simulink model "Projet_RST_sim_LIMA_MILITAO_PINHEIRO"  (R2019a)
settings: Solver=VariableStepAuto  StartTime=0.0  StopTime=10.0  FixedStep=1e-6  RelTol=1e-3
undefined symbols (not defined in the file): Am_omega, Bm_omega, den, G_den_RST, G_num_RST, numG2, R, S, T, Te, tsim
settings Model: Creator=dougl  LastModifiedBy=dougl
settings DebuggingCC: UnconnectedInputMsg=none  UnconnectedOutputMsg=none  UnconnectedLineMsg=none  SFMachineParentedDataDiag=error

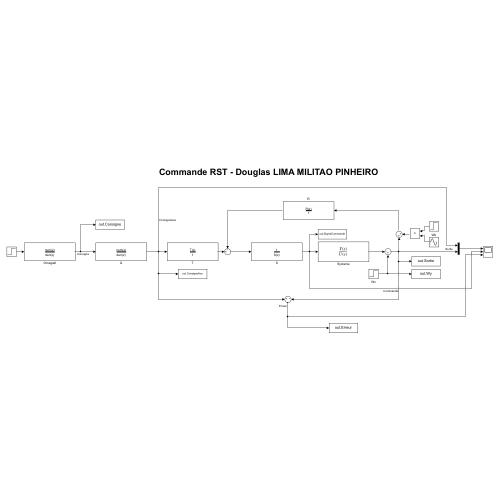
[thumbnail: Simulink's stored preview of the top-level diagram]
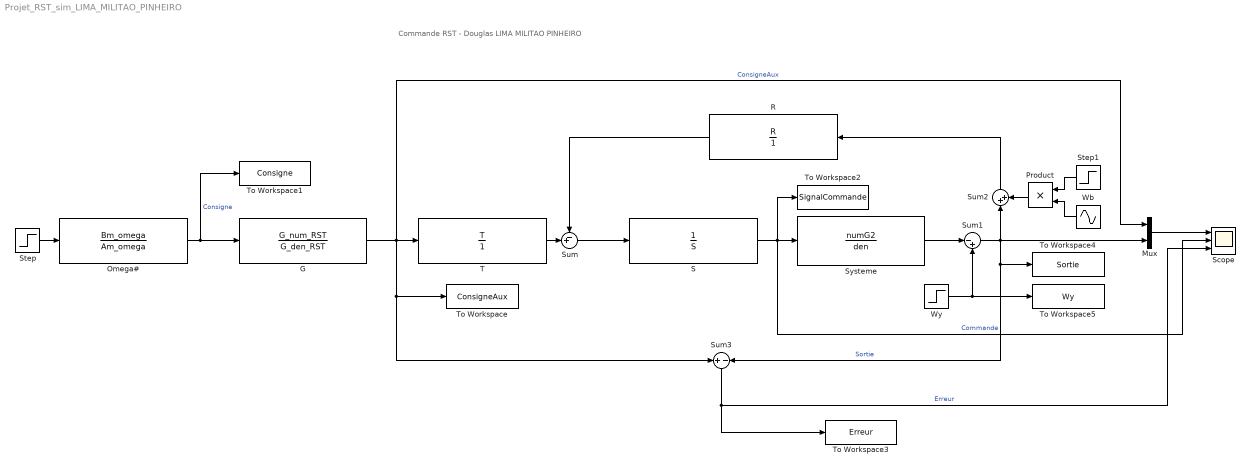
== system Projet_RST_sim_LIMA_MILITAO_PINHEIRO ==
  note: Commande RST - Douglas LIMA MILITAO PINHEIRO
  G : DiscreteFilter  Numerator=G_num_RST  Denominator=G_den_RST  SampleTime=Te
  Mux : Mux  Inputs=2
  Omega# : DiscreteFilter  Numerator=Bm_omega  Denominator=Am_omega  SampleTime=Te
  Product : Product
  R : DiscreteFilter  Numerator=R  Denominator=1  SampleTime=Te
  S : DiscreteFilter  Numerator=1  Denominator=S  SampleTime=Te
  Scope : Scope  NumInputPorts=3
  Step : Step  After=5  SampleTime=0
  Step1 : Step  Time=7  SampleTime=0
  Sum : Sum  Inputs=-+|
  Sum1 : Sum  Inputs=|-+
  Sum2 : Sum  Inputs=|++
  Sum3 : Sum  Inputs=+|-
  Systeme : TransferFcn  Numerator=numG2  Denominator=den
  T : DiscreteFilter  Numerator=T  Denominator=1  SampleTime=Te
  To Workspace : ToWorkspace  VariableName=ConsigneAux  SampleTime=tsim
  To Workspace1 : ToWorkspace  VariableName=Consigne  SampleTime=tsim
  To Workspace2 : ToWorkspace  VariableName=SignalCommande  SampleTime=tsim
  To Workspace3 : ToWorkspace  VariableName=Erreur  SampleTime=tsim
  To Workspace4 : ToWorkspace  VariableName=Sortie  SampleTime=tsim
  To Workspace5 : ToWorkspace  VariableName=Wy  SampleTime=tsim
  Wb : Sin  Amplitude=3  Frequency=2*pi*10  SampleTime=0
  Wy : Step  Time=4  After=15  SampleTime=0
  wires:
  Sum1/1 -> Sum2/1, Mux/2, To Workspace4/1, Sum3/2  "Sortie"
  Sum/1 -> S/1
  Step/1 -> Omega#/1
  T/1 -> Sum/2
  Systeme/1 -> Sum1/1
  Wy/1 -> Sum1/2, To Workspace5/1
  S/1 -> To Workspace2/1, Scope/2, Systeme/1  "Commande"
  Mux/1 -> Scope/1
  R/1 -> Sum/1
  Sum2/1 -> R/1
  G/1 -> Mux/1, T/1, Sum3/1, To Workspace/1  "ConsigneAux"
  Step1/1 -> Product/1
  Wb/1 -> Product/2
  Product/1 -> Sum2/2
  Omega#/1 -> To Workspace1/1, G/1  "Consigne"
  Sum3/1 -> To Workspace3/1, Scope/3  "Erreur"
